simulink model "nonlinearAirframe"  (R2025b)
settings: Solver=ode3  StartTime=0  StopTime=10.0  FixedStep=Ts  RelTol=1e-3  EnableMultiTasking=on
undefined symbols (not defined in the file or in its folder): F, init, Light, MIL, Vehicle
libraries: aerolibasang x1, aerolibwind2 x1
settings Model: Creator=The MathWorks, Inc.  LastModifiedBy=user
settings SolverCC: AlgebraicLoopSolver=TrustRegion
settings DataIOCC: LimitDataPoints=on  SaveFormat=Array  SaveOutput=off  SignalLogging=off  DSMLogging=off  SaveTime=off  ReturnWorkspaceOutputs=off
settings OptimizationCC: BlockReduction=off  DefaultParameterBehavior=Inlined  BufferReuse=off  ReuseModelBlockBuffer=off  LifeSpan=inf
settings DebuggingCC: AlgebraicLoopMsg=none  ParameterPrecisionLossMsg=none  AllowSymbolicDim=off  SFUnexpectedBacktrackingDiag=warning  SFNoUnconditionalDefaultTransitionDiag=warning  SFExecutionAtInitializationDiag=none  ArithmeticOperatorsInVariantConditions=warning
settings HardwareCC: ProdBitPerPointer=32.0  ProdBitPerSizeT=32.0  ProdBitPerPtrDiffT=32.0  ProdLargestAtomicFloat=None  ProdIntDivRoundTo=Undefined  ProdEndianess=Unspecified  ProdWordSize=32.0  ProdHWDeviceType=32-bit Generic
settings ModelReferenceCC: EnableRefExpFcnMdlSchedulingChecks=on  PropagateSignalLabelsOutOfModel=off
settings SFSimCC: SimUseLocalCustomCode=off  CustomCodeUndefinedFunction=UseInterfaceOnly
settings RTWCC: RTWUseLocalCustomCode=off  GPUComputeCapability=3.5
settings CodeAppCC: StateflowObjectComments=on
settings GRTTargetCC: TargetLangStandard=C89/C90 (ANSI)
settings ConfigComp: CovMetricSettings=dw  CovSaveCumulativeToWorkspaceVar=on  CovSaveSingleToWorkspaceVar=on  CovExternalEMLEnable=off  CovSFcnEnable=off

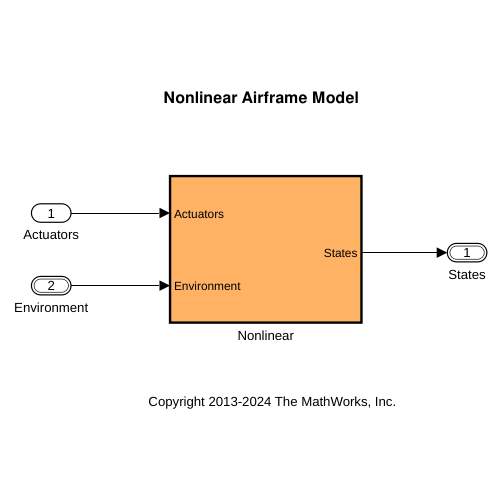
[thumbnail: Simulink's stored preview of the top-level diagram]
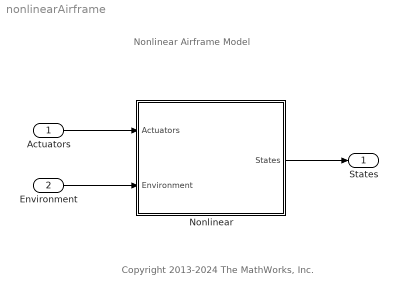
== system nonlinearAirframe ==
  note: Copyright 2013-2024 The MathWorks, Inc.
  note: Nonlinear Airframe Model
  Actuators : Inport  OutDataTypeStr=single  Unit=rpm  PortDimensions=[1 4]
  Environment : Inport  Port=2  OutDataTypeStr=Bus: EnvironmentBus  BusOutputAsStruct=on
  Nonlinear : Subsystem  TreatAsAtomicUnit=on
  States : Outport  OutDataTypeStr=Bus: StatesBus  VectorParamsAs1DForOutWhenUnconnected=off  BusOutputAsStruct=on
  wires:
  Actuators/1 -> Nonlinear/1(Actuators)
  Environment/1 -> Nonlinear/2(Environment)
  Nonlinear/1(States) -> States/1

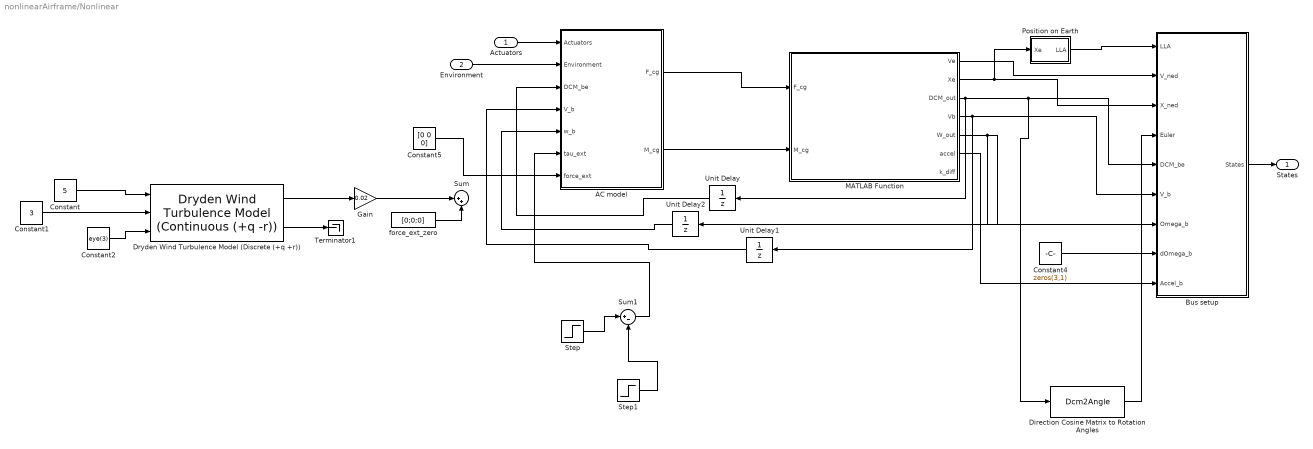
== system nonlinearAirframe/Nonlinear ==
  Actuators : Inport
  Environment : Inport  Port=2
  AC model : Subsystem
  Bus setup : Subsystem
  Constant : Constant  Value=5
  Constant1 : Constant  Value=3
  Constant2 : Constant  Value=eye(3)
  Constant4 : Constant  Value=zeros(3,1)
  Constant5 : Constant  Value=[0 0 0]
  Direction Cosine Matrix to Rotation Angles : Dcm2Angle
      settings: AttributesFormatString=Rotation Order: %<rotationOrder>
  Dryden Wind Turbulence Model (Discrete (+q +r)) : aerolibwind2/Dryden Wind Turbulence Model  (Continuous (+q -r))  units=Metric (MKS)  spec=MIL-F-8785C  model=Discrete Dryden (+q +r)  W20=3  Wdeg=0  TurbProb=10^-2 - Light  L_high=533.4  Wingspan=0.1  ts=0.005  Seed=[23341 23342 23343 23344]  T_on=on
      settings: LibrarySourceBlock=|
      | aerolibwind2/Dryden Wind Turbulence Model
      | (Discrete (+q +r))
  Gain : Gain  Gain=0.02
  MATLAB Function : MATLAB Function  TreatAsAtomicUnit=on
  Position on Earth : Subsystem  Priority=1  TreatAsAtomicUnit=on
  Step : Step  Time=8  Before=[0 0 0]  After=[0 0.24 0]
  Step1 : Step  Time=8.02  Before=[0 0 0]  After=[0 0.24 0]
  Sum : Sum  Inputs=|++
  Sum1 : Sum  Inputs=|+-
  Terminator1 : Terminator
  Unit Delay : UnitDelay  InitialCondition=eye(3)  SampleTime=0.005  HasFrameUpgradeWarning=on
  Unit Delay1 : UnitDelay  InitialCondition=zeros(3,1)  SampleTime=0.005  HasFrameUpgradeWarning=on
  Unit Delay2 : UnitDelay  InitialCondition=zeros(3,1)  SampleTime=0.005  HasFrameUpgradeWarning=on
  force_ext_zero : Constant  Value=[0;0;0]  OutDataTypeStr=double
  States : Outport  VectorParamsAs1DForOutWhenUnconnected=off
  wires:
  Sum1/1 -> AC model/6(tau_ext)
  Constant5/1 -> AC model/7(force_ext)
  Unit Delay2/1 -> AC model/5(w_b)
  Unit Delay1/1 -> AC model/4(V_b)
  Unit Delay/1 -> AC model/3(DCM_be)
  force_ext_zero/1 -> Sum/2
  Gain/1 -> Sum/1
  Dryden Wind Turbulence Model (Discrete (+q +r))/1 -> Gain/1
  Constant2/1 -> Dryden Wind Turbulence Model (Discrete (+q +r))/3
  Constant1/1 -> Dryden Wind Turbulence Model (Discrete (+q +r))/2
  Constant/1 -> Dryden Wind Turbulence Model (Discrete (+q +r))/1
  Dryden Wind Turbulence Model (Discrete (+q +r))/2 -> Terminator1/1
  MATLAB Function/3(DCM_out) -> Direction Cosine Matrix to Rotation Angles/1, Bus setup/5(DCM_be), Unit Delay/1
  MATLAB Function/4(Vb) -> Unit Delay1/1, Bus setup/6(V_b)
  Position on Earth/1(LLA) -> Bus setup/1(LLA)
  Bus setup/1(States) -> States/1
  MATLAB Function/6(accel) -> Bus setup/9(Accel_b)
  Constant4/1 -> Bus setup/8(dOmega_b)
  MATLAB Function/5(W_out) -> Unit Delay2/1, Bus setup/7(Omega_b)
  MATLAB Function/2(Xe) -> Bus setup/3(X_ned), Position on Earth/1(Xe)
  MATLAB Function/1(Ve) -> Bus setup/2(V_ned)
  AC model/2(M_cg) -> MATLAB Function/2(M_cg)
  AC model/1(F_cg) -> MATLAB Function/1(F_cg)
  Environment/1 -> AC model/2(Environment)
  Actuators/1 -> AC model/1(Actuators)
  Step/1 -> Sum1/1
  Step1/1 -> Sum1/2
  Direction Cosine Matrix to Rotation Angles/1 -> Bus setup/4(Euler)

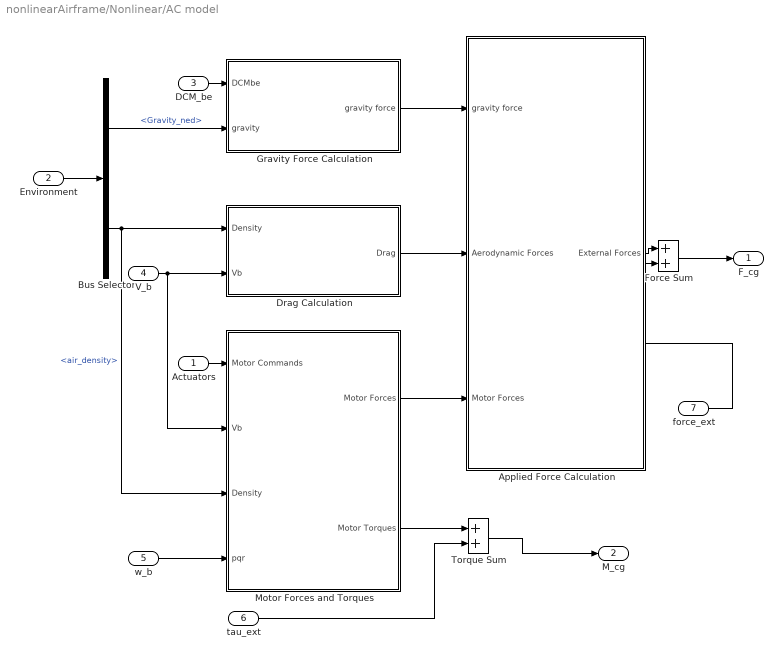
== system nonlinearAirframe/Nonlinear/AC model ==
  Actuators : Inport
  Environment : Inport  Port=2
  DCM_be : Inport  Port=3
  V_b : Inport  Port=4  Unit=m/s
  w_b : Inport  Port=5  Unit=rad/s
  tau_ext : Inport  Port=6  OutDataTypeStr=double  PortDimensions=[3 1]
  force_ext : Inport  Port=7  OutDataTypeStr=double  PortDimensions=[3 1]
  Applied Force Calculation : Subsystem
  Bus Selector : BusSelector  OutputSignals=Gravity_ned,AtmosphereBus.air_density
  Drag Calculation : Subsystem
  Force Sum : Sum
  Gravity Force Calculation : Subsystem
  Motor Forces and Torques : Subsystem
  Torque Sum : Sum
  F_cg : Outport  Unit=N  VectorParamsAs1DForOutWhenUnconnected=off
  M_cg : Outport  Port=2  Unit=N*m  VectorParamsAs1DForOutWhenUnconnected=off
  wires:
  Motor Forces and Torques/1(Motor Forces) -> Applied Force Calculation/3(Motor Forces)
  Bus Selector/1 -> Gravity Force Calculation/2(gravity)  "<Gravity_ned>"
  Gravity Force Calculation/1(gravity force) -> Applied Force Calculation/1(gravity force)
  Environment/1 -> Bus Selector/1
  Bus Selector/2 -> Drag Calculation/1(Density), Motor Forces and Torques/3(Density)  "<air_density>"
  DCM_be/1 -> Gravity Force Calculation/1(DCMbe)
  V_b/1 -> Drag Calculation/2(Vb), Motor Forces and Torques/2(Vb)
  Drag Calculation/1(Drag) -> Applied Force Calculation/2(Aerodynamic Forces)
  Actuators/1 -> Motor Forces and Torques/1(Motor Commands)
  w_b/1 -> Motor Forces and Torques/4(pqr)
  Motor Forces and Torques/2(Motor Torques) -> Torque Sum/1
  tau_ext/1 -> Torque Sum/2
  Torque Sum/1 -> M_cg/1
  Applied Force Calculation/1(External Forces) -> Force Sum/1
  force_ext/1 -> Force Sum/2
  Force Sum/1 -> F_cg/1

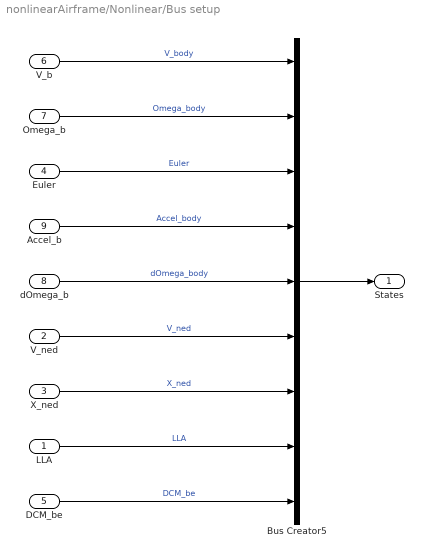
== system nonlinearAirframe/Nonlinear/Bus setup ==
  LLA : Inport  PortDimensions=3
  V_ned : Inport  Port=2  Unit=m/second  PortDimensions=3
  X_ned : Inport  Port=3  Unit=m  PortDimensions=3
  Euler : Inport  Port=4  Unit=rad  PortDimensions=3
  DCM_be : Inport  Port=5  PortDimensions=[3 3]
  V_b : Inport  Port=6  Unit=m/s  PortDimensions=3
  Omega_b : Inport  Port=7  Unit=rad/s  PortDimensions=3
  dOmega_b : Inport  Port=8  Unit=rad/s^2  PortDimensions=3
  Accel_b : Inport  Port=9  Unit=m/s^2  PortDimensions=3
  Bus Creator5 : BusCreator  Inputs=9  OutDataTypeStr=Bus: StatesBus  NonVirtualBus=on
  States : Outport  VectorParamsAs1DForOutWhenUnconnected=off
  wires:
  Bus Creator5/1 -> States/1
  V_b/1 -> Bus Creator5/1  "V_body"
  Omega_b/1 -> Bus Creator5/2  "Omega_body"
  Euler/1 -> Bus Creator5/3  "Euler"
  X_ned/1 -> Bus Creator5/7  "X_ned"
  Accel_b/1 -> Bus Creator5/4  "Accel_body"
  LLA/1 -> Bus Creator5/8  "LLA"
  dOmega_b/1 -> Bus Creator5/5  "dOmega_body"
  DCM_be/1 -> Bus Creator5/9  "DCM_be"
  V_ned/1 -> Bus Creator5/6  "V_ned"

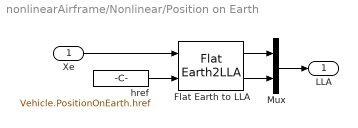
== system nonlinearAirframe/Nonlinear/Position on Earth ==
  Xe : Inport  Unit=m
  Flat Earth to LLA : FlatEarth2LLA  R=6378137  LL0=init.posLLA(1:2)  psi=Vehicle.PositionOnEarth.FlatEarthToLLA.xAxis
  Mux : Mux  Inputs=2
  href : Constant  Value=Vehicle.PositionOnEarth.href
  LLA : Outport  VectorParamsAs1DForOutWhenUnconnected=off
  wires:
  Mux/1 -> LLA/1
  Xe/1 -> Flat Earth to LLA/1
  Flat Earth to LLA/1 -> Mux/1
  Flat Earth to LLA/2 -> Mux/2
  href/1 -> Flat Earth to LLA/2

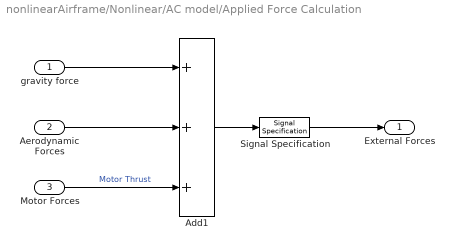
== system nonlinearAirframe/Nonlinear/AC model/Applied Force Calculation ==
  gravity force : Inport  Unit=N
  Aerodynamic Forces : Inport  Port=2  Unit=N
  Motor Forces : Inport  Port=3  Unit=N
  Add1 : Sum  Inputs=+++
  Signal Specification : SignalSpecification  Dimensions=3
  External Forces : Outport  Unit=N  VectorParamsAs1DForOutWhenUnconnected=off
  wires:
  Add1/1 -> Signal Specification/1
  Motor Forces/1 -> Add1/3  "Motor Thrust"
  Aerodynamic Forces/1 -> Add1/2
  gravity force/1 -> Add1/1
  Signal Specification/1 -> External Forces/1

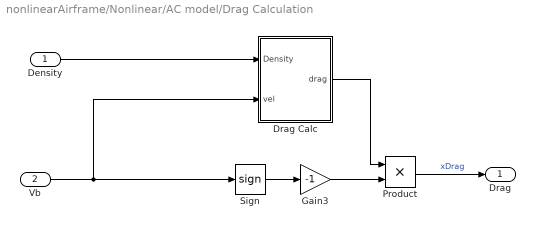
== system nonlinearAirframe/Nonlinear/AC model/Drag Calculation ==
  Density : Inport  Unit=kg/m^3
  Vb : Inport  Port=2  Unit=m/second
  Drag Calc : Subsystem
  Gain3 : Gain  Gain=-1
  Product : Product  RndMeth=Zero
  Sign : Signum  ZeroCross=off
  Drag : Outport  Unit=N  VectorParamsAs1DForOutWhenUnconnected=off
  wires:
  Density/1 -> Drag Calc/1(Density)
  Sign/1 -> Gain3/1
  Drag Calc/1(drag) -> Product/1
  Gain3/1 -> Product/2
  Product/1 -> Drag/1  "xDrag"
  Vb/1 -> Sign/1, Drag Calc/2(vel)

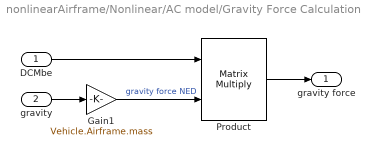
== system nonlinearAirframe/Nonlinear/AC model/Gravity Force Calculation ==
  DCMbe : Inport
  gravity : Inport  Port=2  Unit=m/s^2
  Gain1 : Gain  Gain=Vehicle.Airframe.mass
  Product : Product  Multiplication=Matrix(*)
  gravity force : Outport  Unit=N  VectorParamsAs1DForOutWhenUnconnected=off
  wires:
  gravity/1 -> Gain1/1
  Gain1/1 -> Product/2  "gravity force NED"
  Product/1 -> gravity force/1
  DCMbe/1 -> Product/1

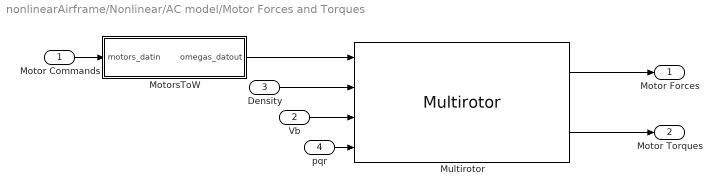
== system nonlinearAirframe/Nonlinear/AC model/Motor Forces and Torques ==
  Motor Commands : Inport
  Vb : Inport  Port=2
  Density : Inport  Port=3
  pqr : Inport  Port=4
  MotorsToW : Subsystem
  Multirotor : Multirotor  modelMode=With flap effects  armLength=Vehicle.Airframe.d  rotorHeight=Vehicle.Airframe.h  CT=Vehicle.Rotor.Ct  CQ=Vehicle.Rotor.Cq  Nb=Vehicle.Rotor.blades  radius=Vehicle.Rotor.radius  chord=Vehicle.Rotor.chord  hingeOffset=Vehicle.Rotor.flappingOffset  clalpha=Vehicle.Rotor.a  gamma=Vehicle.Rotor.lock  thetaRoot=Vehicle.Rotor.theta0  thetaTwist=Vehicle.Rotor.theta1
      settings: LibrarySourceBlock=aerolibrotor/Rotor
  Motor Forces : Outport  Unit=N  VectorParamsAs1DForOutWhenUnconnected=off
  Motor Torques : Outport  Port=2  Unit=N*m  VectorParamsAs1DForOutWhenUnconnected=off
  wires:
  MotorsToW/1(omegas_datout) -> Multirotor/1
  pqr/1 -> Multirotor/4
  Vb/1 -> Multirotor/3
  Motor Commands/1 -> MotorsToW/1(motors_datin)
  Density/1 -> Multirotor/2
  Multirotor/1 -> Motor Forces/1
  Multirotor/2 -> Motor Torques/1

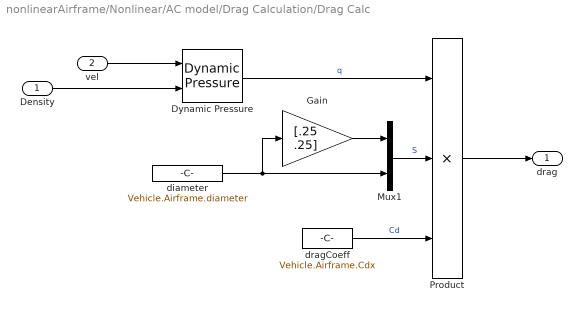
== system nonlinearAirframe/Nonlinear/AC model/Drag Calculation/Drag Calc ==
  Density : Inport  Unit=kg/m^3
  vel : Inport  Port=2  Unit=m/s
  Dynamic Pressure : aerolibasang/Dynamic Pressure
  Gain : Gain  Gain=[.25 .25]
  Mux1 : Mux  Inputs=2
  Product : Product  Inputs=3  RndMeth=Zero
  diameter : Constant  Value=Vehicle.Airframe.diameter  SampleTime=0
  dragCoeff : Constant  Value=Vehicle.Airframe.Cdx  SampleTime=0
  drag : Outport  Unit=N  VectorParamsAs1DForOutWhenUnconnected=off
  wires:
  Product/1 -> drag/1
  dragCoeff/1 -> Product/3  "Cd"
  Dynamic Pressure/1 -> Product/1  "q"
  diameter/1 -> Gain/1, Mux1/2
  Mux1/1 -> Product/2  "S"
  Gain/1 -> Mux1/1
  vel/1 -> Dynamic Pressure/1
  Density/1 -> Dynamic Pressure/2

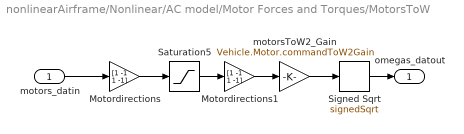
== system nonlinearAirframe/Nonlinear/AC model/Motor Forces and Torques/MotorsToW ==
  motors_datin : Inport
  Motordirections : Gain  Gain=[1 -1 1 -1]  ParamDataTypeStr=single  OutDataTypeStr=Inherit: Inherit via back propagation  SaturateOnIntegerOverflow=on
  Motordirections1 : Gain  Gain=[1 -1 1 -1]  ParamDataTypeStr=single  OutDataTypeStr=Inherit: Inherit via back propagation  SaturateOnIntegerOverflow=on
  Saturation5 : Saturate  UpperLimit=Vehicle.Motor.maxLimit  LowerLimit=Vehicle.Motor.minLimit  OutDataTypeStr=Inherit: Inherit via back propagation
  Signed Sqrt : Sqrt  Operator=signedSqrt  OutDataTypeStr=Inherit: Inherit via back propagation
  motorsToW2_Gain : Gain  Gain=Vehicle.Motor.commandToW2Gain  ParamDataTypeStr=single  OutDataTypeStr=Inherit: Inherit via back propagation  SaturateOnIntegerOverflow=on
  omegas_datout : Outport  VectorParamsAs1DForOutWhenUnconnected=off
  wires:
  motorsToW2_Gain/1 -> Signed Sqrt/1
  Motordirections/1 -> Saturation5/1
  Saturation5/1 -> Motordirections1/1
  Motordirections1/1 -> motorsToW2_Gain/1
  Signed Sqrt/1 -> omegas_datout/1
  motors_datin/1 -> Motordirections/1

== matlab function nonlinearAirframe/Nonlinear/MATLAB Function ==
  data: F_cg input double size=[3 1]; Ve output double size=[3 1]; M_cg input double size=[3 1]; Xe output double size=[3 1]; DCM_out output double size=[3 3]; Vb output double size=[3 1]; W_out output double size=[3 1]; accel output double size=[3 1]; k_diff output
function [Ve, Xe, DCM_out, Vb, W_out, accel, k_diff] = SO3_dynamics(F_cg, M_cg)

persistent Cbe W xN vN k_history

% 초기조건
if isempty(Cbe)
    Cbe = eye(3);
    W   = zeros(3,1);
    xN  = [57; 95; -0.046];
    vN  = zeros(3,1);
    k_history = [];
end

% 드론 스펙 및 환경

m  = 0.063;
J  = diag([5.82857e-5, 7.16914e-5, 1e-4]);
dt = 0.005;
ground_z = -0.046;

F = reshape(double(F_cg), 3, 1);
M = reshape(double(M_cg), 3, 1);

% 이전 속도 저장
vN_prev = vN;

% body-axis force -> inertial/NED acceleration
% a = F/m
aN = Cbe.' * (F ./ m);      % F = body frame , aN = NED frame , Cbe = body -> NED 변환

% translational integration
% velocity and position by accel integration

vN = vN + dt .* aN;
xN = xN + dt .* vN;

% ground constraint
on_ground = (xN(3) >= ground_z);

if on_ground
    xN(3) = ground_z;

    % NED 기준: +z는 아래 방향. 바닥으로 파고드는 속도 제거
    if vN(3) > 0
        vN(3) = 0;
    end

end


% rotational dynamics

k1 = J \ (M - cross(W,          J*W));
k2 = J \ (M - cross(W+dt/2*k1, J*(W+dt/2*k1)));
k3 = J \ (M - cross(W+dt/2*k2, J*(W+dt/2*k2)));
k4 = J \ (M - cross(W+dt*k3,   J*(W+dt*k3)));
Wmid = W + dt/2 .* k1;                          % k1 계산 후에 midpoint 구함
W    = W + dt/6 .* (k1 + 2*k2 + 2*k3 + k4);


% k1을 기준으로 각 단계별 벡터가 얼마나 벌어지는지 '크기(Norm)' 계산
k1_norm = norm(k1);
diff_k2 = norm(k2 - k1);
diff_k3 = norm(k3 - k1);
diff_k4 = norm(k4 - k1);

% 타임스텝마다 가로로 쌓기
k_history = [k_history; k1_norm, diff_k2, diff_k3, diff_k4];

% attitude update
Cbe = expSO3(-Wmid .* dt) * Cbe;     % SO(3) 곱셈으로 처리 + 크기 1로 유지
Cbe = normalizeDCM(Cbe);

% outputs
Ve      = vN;
Xe      = xN;
DCM_out = Cbe;
Vb      = Cbe * vN;
W_out   = W;
accel   =  F ./ m;
k_diff  = [k1_norm; diff_k2; diff_k3; diff_k4];
end

function S = hat3(w)
S = [0, -w(3), w(2); w(3), 0, -w(1); -w(2), w(1), 0];
end

function R = expSO3(phi)
theta = sqrt(phi(1)*phi(1) + phi(2)*phi(2) + phi(3)*phi(3));
K = hat3(phi);
if theta < 1e-9
    R = eye(3) + K + 0.5 .* (K*K);
else
    a = sin(theta) ./ theta;
    b = (1 - cos(theta)) ./ (theta .* theta);
    R = eye(3) + a .* K + b .* (K*K);
end
end

function C = normalizeDCM(Cin)
x = Cin(:,1);
y = Cin(:,2);
x = x ./ sqrt(x.'*x);
y = y - x .* (x.'*y);
y = y ./ sqrt(y.'*y);
z = cross(x,y);
C = [x, y, z];
end
